simulink model "rst_auto_reg_coupled_tanks_cascade_2018b"  (R2018b)
settings: Solver=FixedStepAuto  StartTime=0.0  StopTime=1000  FixedStep=0.1  RelTol=1e-3
InitFcn:
  | g = 981
  | Km = 3.3
  | Ao1 = 0.17
  | At1 = 15.5528
  | Ao2 = 0.17
  | At2 = 15.5528
  | Ta = 0.1
  | initial_theta = [rand(1,2)]
libraries: dspinverses x4
settings Model: Creator=root  LastModifiedBy=root
settings DataIOCC: SaveFormat=StructureWithTime
settings OptimizationCC: LifeSpan=inf
settings DebuggingCC: LibraryContextMissingDiagnostic=none  SFExecutionAtInitializationDiag=none
settings HardwareCC: ProdBitPerSizeT=32  ProdBitPerPtrDiffT=32  ProdWordSize=32  ProdHWDeviceType=Specified
settings CodeAppCC: StateflowObjectComments=on

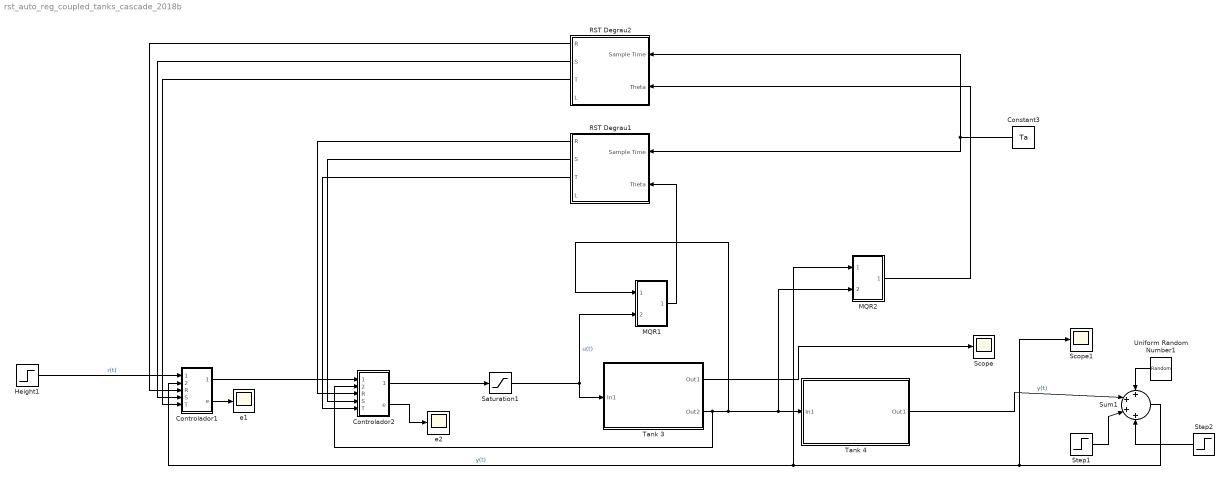
== system rst_auto_reg_coupled_tanks_cascade_2018b ==
  Constant3 : Constant  Value=Ta
  Controlador1 : Subsystem
  Controlador2 : Subsystem
  Height1 : Step  Time=0  After=10  SampleTime=0
  MQR1 : Subsystem
  MQR2 : Subsystem
  RST Degrau1 : Subsystem
  RST Degrau2 : Subsystem
  Saturation1 : Saturate  UpperLimit=12  LowerLimit=-12
  Scope : Scope
  Scope1 : Scope
  Step1 : Step  Time=60  SampleTime=0
  Step2 : Step  Time=61  After=-1  SampleTime=0
  Sum1 : Sum  Inputs=++++
  Tank 3 : Subsystem
  Tank 4 : Subsystem
  Uniform Random Number1 : UniformRandomNumber  Minimum=-0.05  Maximum=0.05  SampleTime=0
  e1 : Scope
  e2 : Scope
  wires:
  Saturation1/1 -> Tank 3/1(In1), MQR1/2("u(t) ")  "u(t)"
  Uniform Random Number1/1 -> Sum1/1
  Step2/1 -> Sum1/4
  Step1/1 -> Sum1/3
  Tank 4/1(Out1) -> Sum1/2  "y(t)"
  Sum1/1 -> Scope1/1, MQR2/1(y(t)), Controlador1/2(y(t))  "y(t)"
  Controlador1/1(u(t)) -> Controlador2/1(r(t))
  Tank 3/2(Out2) -> Controlador2/2(y(t)), MQR1/1(y(t)), MQR2/2("u(t) "), Tank 4/1(In1)
  MQR1/1("Theta(t) ") -> RST Degrau1/2(Theta)
  RST Degrau1/1(R) -> Controlador2/3(R)
  RST Degrau1/2(S) -> Controlador2/4(S)
  RST Degrau1/3(T) -> Controlador2/5(T)
  MQR2/1("Theta(t) ") -> RST Degrau2/2(Theta)
  RST Degrau2/1(R) -> Controlador1/3(R)
  RST Degrau2/2(S) -> Controlador1/4(S)
  RST Degrau2/3(T) -> Controlador1/5(T)
  Height1/1 -> Controlador1/1(r(t))  "r(t)"
  Controlador2/2("e ") -> e2/1
  Controlador2/1(u(t)) -> Saturation1/1
  Controlador1/2("e ") -> e1/1
  Constant3/1 -> RST Degrau1/1(Sample Time), RST Degrau2/1(Sample Time)
  Tank 3/1(Out1) -> Scope/1

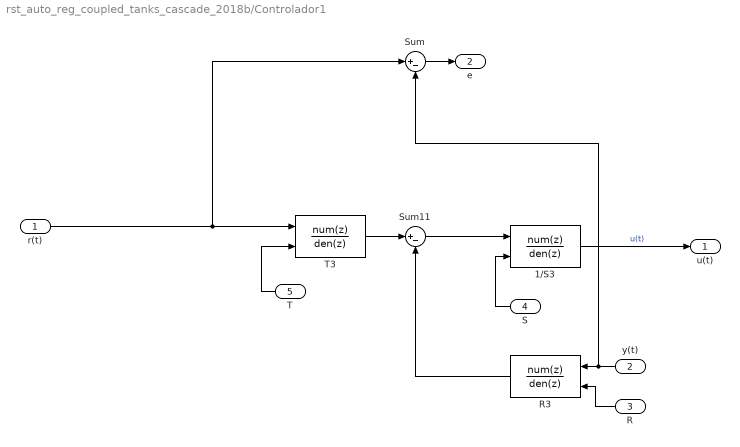
== system rst_auto_reg_coupled_tanks_cascade_2018b/Controlador1 ==
  r(t) : Inport
  y(t) : Inport  Port=2
  R : Inport  Port=3
  S : Inport  Port=4
  T : Inport  Port=5
  1/S3 : DiscreteFilter  Numerator=1  DenominatorSource=Input port  Denominator=1  SampleTime=Ta  a0EqualsOne=on
      settings: InputPortMap=u0,p3
  R3 : DiscreteFilter  NumeratorSource=Input port  Numerator=[-620.2 131.3]  Denominator=1  SampleTime=Ta
      settings: InputPortMap=u0,p1
  Sum : Sum  Inputs=|+-
  Sum11 : Sum  Inputs=|+-
  T3 : DiscreteFilter  NumeratorSource=Input port  Numerator=13.39  Denominator=1  SampleTime=Ta
      settings: InputPortMap=u0,p1
  u(t) : Outport
  "e " : Outport  Port=2
  wires:
  Sum/1 -> "e "/1
  1/S3/1 -> u(t)/1  "u(t)"
  T/1 -> T3/2
  r(t)/1 -> T3/1, Sum/1
  S/1 -> 1/S3/2
  y(t)/1 -> R3/1, Sum/2
  T3/1 -> Sum11/1
  Sum11/1 -> 1/S3/1
  R3/1 -> Sum11/2
  R/1 -> R3/2

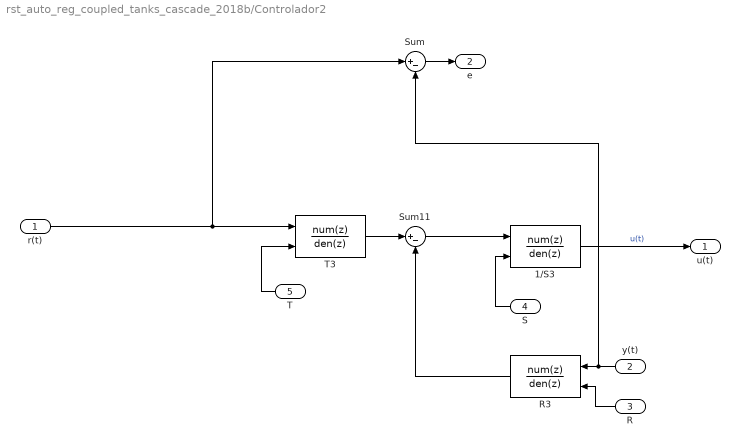
== system rst_auto_reg_coupled_tanks_cascade_2018b/Controlador2 ==
  r(t) : Inport
  y(t) : Inport  Port=2
  R : Inport  Port=3
  S : Inport  Port=4
  T : Inport  Port=5
  1/S3 : DiscreteFilter  Numerator=1  DenominatorSource=Input port  Denominator=1  SampleTime=Ta  a0EqualsOne=on
      settings: InputPortMap=u0,p3
  R3 : DiscreteFilter  NumeratorSource=Input port  Numerator=[-620.2 131.3]  Denominator=1  SampleTime=Ta
      settings: InputPortMap=u0,p1
  Sum : Sum  Inputs=|+-
  Sum11 : Sum  Inputs=|+-
  T3 : DiscreteFilter  NumeratorSource=Input port  Numerator=13.39  Denominator=1  SampleTime=Ta
      settings: InputPortMap=u0,p1
  u(t) : Outport
  "e " : Outport  Port=2
  wires:
  R/1 -> R3/2
  R3/1 -> Sum11/2
  Sum11/1 -> 1/S3/1
  T3/1 -> Sum11/1
  y(t)/1 -> Sum/2, R3/1
  S/1 -> 1/S3/2
  r(t)/1 -> Sum/1, T3/1
  T/1 -> T3/2
  1/S3/1 -> u(t)/1  "u(t)"
  Sum/1 -> "e "/1

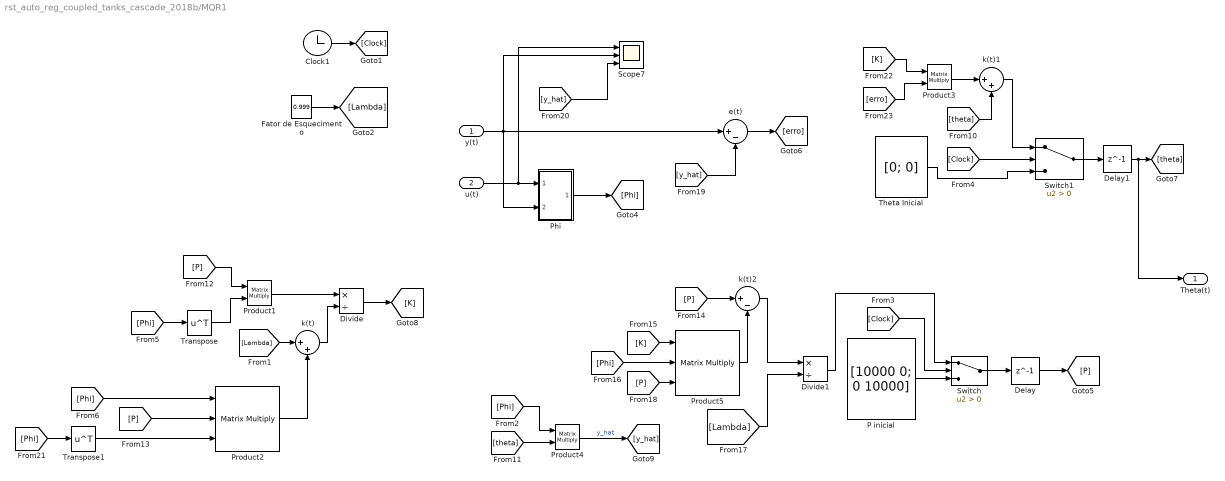
== system rst_auto_reg_coupled_tanks_cascade_2018b/MQR1 ==
  y(t) : Inport
  "u(t) " : Inport  Port=2
  Clock1 : Clock
  Delay : Delay  DelayLength=1  InitialCondition=0
  Delay1 : Delay  DelayLength=1  InitialCondition=0
  Divide : Product  Inputs=*/
  Divide1 : Product  Inputs=*/
  "Fator de Esquecimento " : Constant  Value=0.999
  P inicial : Constant  Value=[10000 0; 0 10000]
  Phi : Subsystem
  Product1 : Product  Multiplication=Matrix(*)
  Product2 : Product  Inputs=3  Multiplication=Matrix(*)
  Product3 : Product  Multiplication=Matrix(*)
  Product4 : Product  Multiplication=Matrix(*)
  Product5 : Product  Inputs=3  Multiplication=Matrix(*)
  Scope7 : Scope  NumInputPorts=3
  Switch : Switch  Criteria=u2 > Threshold
  Switch1 : Switch  Criteria=u2 > Threshold
  "Theta Inicial " : Constant  Value=[0; 0]
  Transpose : Math  Operator=transpose  SaturateOnIntegerOverflow=on
  Transpose1 : Math  Operator=transpose  SaturateOnIntegerOverflow=on
  e(t) : Sum  Inputs=|+-
  k(t) : Sum  Inputs=|++
  k(t)1 : Sum  Inputs=|++
  k(t)2 : Sum  Inputs=|+-
  "Theta(t) " : Outport
  wires:
  Product4/1 -> [y_hat]  "y_hat"
  [Phi] -> Product5/2
  Divide/1 -> [K]
  [Phi] -> Product2/1
  [P] -> Product1/1
  P inicial/1 -> Switch/3
  [K] -> Product5/1
  [y_hat] -> e(t)/2
  [erro] -> Product3/2
  Clock1/1 -> [Clock]
  Transpose/1 -> Product1/2
  [Lambda] -> k(t)/1
  [P] -> Product2/2
  [theta] -> k(t)1/2
  [P] -> k(t)2/1
  [theta] -> Product4/2
  [Clock] -> Switch/2
  [Phi] -> Transpose/1
  Divide1/1 -> Switch/1
  Transpose1/1 -> Product2/3
  "Theta Inicial "/1 -> Switch1/3
  "Fator de Esquecimento "/1 -> [Lambda]
  [P] -> Product5/3
  [Phi] -> Transpose1/1
  Delay/1 -> [P]
  Product3/1 -> k(t)1/1
  e(t)/1 -> [erro]
  Product1/1 -> Divide/1
  [Lambda] -> Divide1/2
  Switch/1 -> Delay/1
  "u(t) "/1 -> Phi/1(u(t)), Scope7/1
  Product5/1 -> k(t)2/2
  Delay1/1 -> [theta], "Theta(t) "/1
  k(t)2/1 -> Divide1/1
  y(t)/1 -> Phi/2(y(t)), Scope7/2, e(t)/1
  [Clock] -> Switch1/2
  Product2/1 -> k(t)/2
  [K] -> Product3/1
  Switch1/1 -> Delay1/1
  [y_hat] -> Scope7/3
  k(t)1/1 -> Switch1/1
  Phi/1(Phi) -> [Phi]
  [Phi] -> Product4/1
  k(t)/1 -> Divide/2

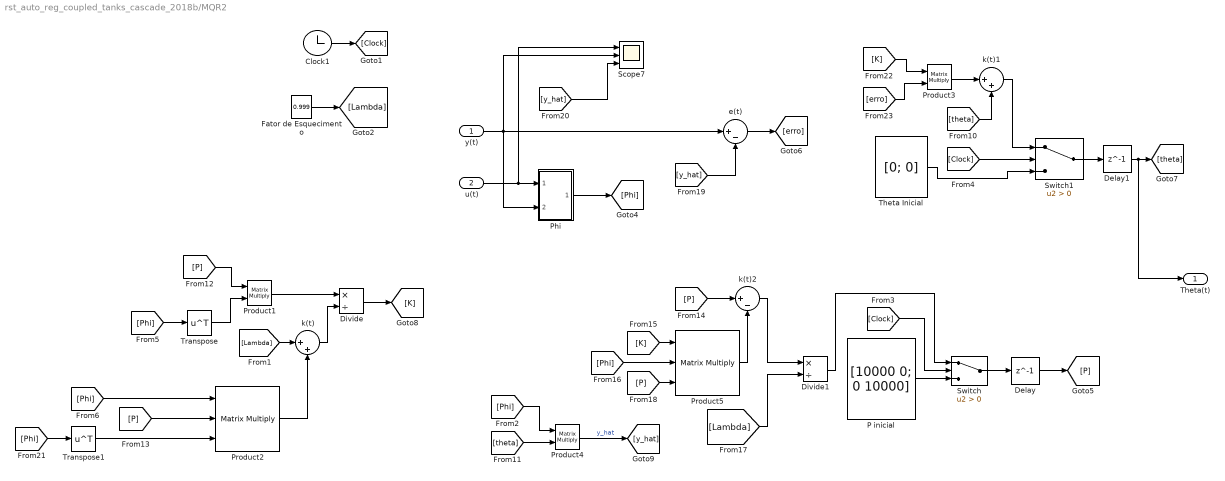
== system rst_auto_reg_coupled_tanks_cascade_2018b/MQR2 ==
  y(t) : Inport
  "u(t) " : Inport  Port=2
  Clock1 : Clock
  Delay : Delay  DelayLength=1  InitialCondition=0
  Delay1 : Delay  DelayLength=1  InitialCondition=0
  Divide : Product  Inputs=*/
  Divide1 : Product  Inputs=*/
  "Fator de Esquecimento " : Constant  Value=0.999
  P inicial : Constant  Value=[10000 0; 0 10000]
  Phi : Subsystem
  Product1 : Product  Multiplication=Matrix(*)
  Product2 : Product  Inputs=3  Multiplication=Matrix(*)
  Product3 : Product  Multiplication=Matrix(*)
  Product4 : Product  Multiplication=Matrix(*)
  Product5 : Product  Inputs=3  Multiplication=Matrix(*)
  Scope7 : Scope  NumInputPorts=3
  Switch : Switch  Criteria=u2 > Threshold
  Switch1 : Switch  Criteria=u2 > Threshold
  "Theta Inicial " : Constant  Value=[0; 0]
  Transpose : Math  Operator=transpose  SaturateOnIntegerOverflow=on
  Transpose1 : Math  Operator=transpose  SaturateOnIntegerOverflow=on
  e(t) : Sum  Inputs=|+-
  k(t) : Sum  Inputs=|++
  k(t)1 : Sum  Inputs=|++
  k(t)2 : Sum  Inputs=|+-
  "Theta(t) " : Outport
  wires:
  k(t)/1 -> Divide/2
  [Phi] -> Product4/1
  Phi/1(Phi) -> [Phi]
  k(t)1/1 -> Switch1/1
  [y_hat] -> Scope7/3
  Switch1/1 -> Delay1/1
  [K] -> Product3/1
  Product2/1 -> k(t)/2
  [Clock] -> Switch1/2
  y(t)/1 -> e(t)/1, Scope7/2, Phi/2(y(t))
  k(t)2/1 -> Divide1/1
  Delay1/1 -> "Theta(t) "/1, [theta]
  Product5/1 -> k(t)2/2
  "u(t) "/1 -> Scope7/1, Phi/1(u(t))
  Switch/1 -> Delay/1
  [Lambda] -> Divide1/2
  Product1/1 -> Divide/1
  e(t)/1 -> [erro]
  Product3/1 -> k(t)1/1
  Delay/1 -> [P]
  [Phi] -> Transpose1/1
  [P] -> Product5/3
  "Fator de Esquecimento "/1 -> [Lambda]
  "Theta Inicial "/1 -> Switch1/3
  Transpose1/1 -> Product2/3
  Divide1/1 -> Switch/1
  [Phi] -> Transpose/1
  [Clock] -> Switch/2
  [theta] -> Product4/2
  [P] -> k(t)2/1
  [theta] -> k(t)1/2
  [P] -> Product2/2
  [Lambda] -> k(t)/1
  Transpose/1 -> Product1/2
  Clock1/1 -> [Clock]
  [erro] -> Product3/2
  [y_hat] -> e(t)/2
  [K] -> Product5/1
  P inicial/1 -> Switch/3
  [P] -> Product1/1
  [Phi] -> Product2/1
  Divide/1 -> [K]
  [Phi] -> Product5/2
  Product4/1 -> [y_hat]  "y_hat"

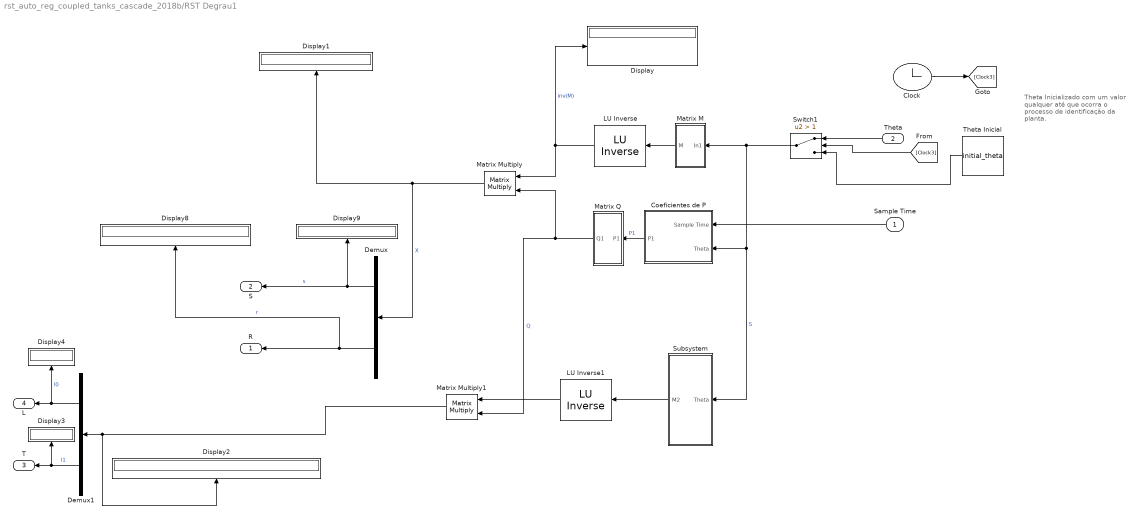
== system rst_auto_reg_coupled_tanks_cascade_2018b/RST Degrau1 ==
  note: Theta Inicializado com um
      | valor qualquer até que ocorra
      |  o processo de identificação
      | da planta.
  Sample Time : Inport
  Theta : Inport  Port=2
  " LU Inverse" : dspinverses/ LU Inverse
      settings: SourceProductName=DSP System Toolbox
  " LU Inverse1" : dspinverses/ LU Inverse
      settings: SourceProductName=DSP System Toolbox
  Clock : Clock
  Coeficientes de P : Subsystem
  Demux : Demux  Outputs=2
  Demux1 : Demux  Outputs=2
  Display{,1..4,8..9} (7 alike) : Display
  Matrix M : Subsystem
  Matrix Multiply : Product  Multiplication=Matrix(*)
  Matrix Multiply1 : Product  Multiplication=Matrix(*)
  Matrix Q : Subsystem
  Subsystem : Subsystem
  Switch1 : Switch  Criteria=u2 > Threshold  Threshold=1
  Theta Inicial : Constant  Value=initial_theta
  R : Outport
  S : Outport  Port=2
  T : Outport  Port=3
  L : Outport  Port=4
  wires:
  Demux/2 -> R/1, Display8/1  "r"
  Demux1/2 -> T/1, Display3/1  "l1"
  Matrix Multiply1/1 -> Demux1/1, Display2/1
  Demux1/1 -> Display4/1, L/1  "l0"
  Subsystem/1(M2) -> " LU Inverse1"/1
  Matrix Q/1(Q1) -> Matrix Multiply/2, Matrix Multiply1/2  "Q"
  " LU Inverse1"/1 -> Matrix Multiply1/1
  Demux/1 -> S/1, Display9/1  "s"
  Matrix M/1(M) -> " LU Inverse"/1
  Theta Inicial/1 -> Switch1/3
  [Clock3] -> Switch1/2
  Theta/1 -> Switch1/1
  Switch1/1 -> Matrix M/1(In1), Subsystem/1(Theta), Coeficientes de P/2(Theta)  "S"
  Clock/1 -> [Clock3]
  Coeficientes de P/1(P1) -> Matrix Q/1(P1)  "P1"
  Sample Time/1 -> Coeficientes de P/1(Sample Time)
  " LU Inverse"/1 -> Display/1, Matrix Multiply/1  "inv(M)"
  Matrix Multiply/1 -> Display1/1, Demux/1  "X"

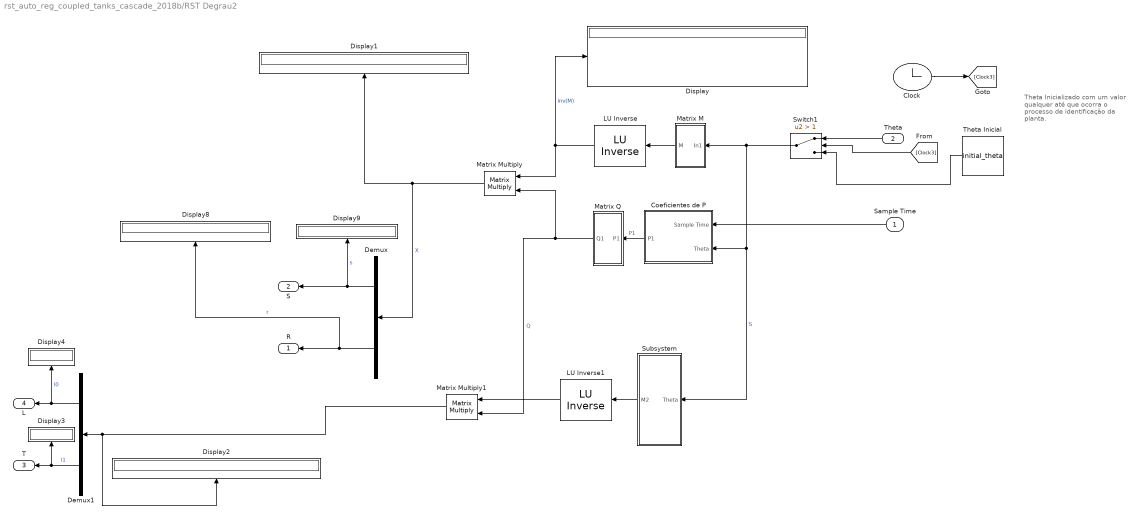
== system rst_auto_reg_coupled_tanks_cascade_2018b/RST Degrau2 ==
  note: Theta Inicializado com um
      | valor qualquer até que ocorra
      |  o processo de identificação
      | da planta.
  Sample Time : Inport
  Theta : Inport  Port=2
  " LU Inverse" : dspinverses/ LU Inverse
      settings: SourceProductName=DSP System Toolbox
  " LU Inverse1" : dspinverses/ LU Inverse
      settings: SourceProductName=DSP System Toolbox
  Clock : Clock
  Coeficientes de P : Subsystem
  Demux : Demux  Outputs=2
  Demux1 : Demux  Outputs=2
  Display{,1..4,8..9} (7 alike) : Display
  Matrix M : Subsystem
  Matrix Multiply : Product  Multiplication=Matrix(*)
  Matrix Multiply1 : Product  Multiplication=Matrix(*)
  Matrix Q : Subsystem
  Subsystem : Subsystem
  Switch1 : Switch  Criteria=u2 > Threshold  Threshold=1
  Theta Inicial : Constant  Value=initial_theta
  R : Outport
  S : Outport  Port=2
  T : Outport  Port=3
  L : Outport  Port=4
  wires:
  Matrix Multiply/1 -> Demux/1, Display1/1  "X"
  " LU Inverse"/1 -> Matrix Multiply/1, Display/1  "inv(M)"
  Sample Time/1 -> Coeficientes de P/1(Sample Time)
  Coeficientes de P/1(P1) -> Matrix Q/1(P1)  "P1"
  Clock/1 -> [Clock3]
  Switch1/1 -> Subsystem/1(Theta), Coeficientes de P/2(Theta), Matrix M/1(In1)  "S"
  Theta/1 -> Switch1/1
  [Clock3] -> Switch1/2
  Theta Inicial/1 -> Switch1/3
  Matrix M/1(M) -> " LU Inverse"/1
  Demux/1 -> S/1, Display9/1  "s"
  " LU Inverse1"/1 -> Matrix Multiply1/1
  Matrix Q/1(Q1) -> Matrix Multiply1/2, Matrix Multiply/2  "Q"
  Subsystem/1(M2) -> " LU Inverse1"/1
  Demux1/1 -> L/1, Display4/1  "l0"
  Matrix Multiply1/1 -> Display2/1, Demux1/1
  Demux1/2 -> Display3/1, T/1  "l1"
  Demux/2 -> R/1, Display8/1  "r"

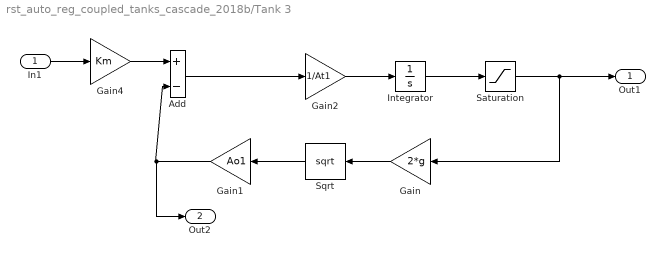
== system rst_auto_reg_coupled_tanks_cascade_2018b/Tank 3 ==
  In1 : Inport
  Add : Sum  Inputs=+-
  Gain : Gain  Gain=2*g
  Gain1 : Gain  Gain=Ao1
  Gain2 : Gain  Gain=1/At1
  Gain4 : Gain  Gain=Km
  Integrator : Integrator
  Saturation : Saturate  UpperLimit=30  LowerLimit=0
  Sqrt : Sqrt  SaturateOnIntegerOverflow=on
  Out1 : Outport
  Out2 : Outport  Port=2
  wires:
  Gain4/1 -> Add/1
  Add/1 -> Gain2/1
  Saturation/1 -> Gain/1, Out1/1
  Integrator/1 -> Saturation/1
  Sqrt/1 -> Gain1/1
  In1/1 -> Gain4/1
  Gain/1 -> Sqrt/1
  Gain1/1 -> Add/2, Out2/1
  Gain2/1 -> Integrator/1

== system rst_auto_reg_coupled_tanks_cascade_2018b/Tank 4 ==
  In1 : Inport
  Add1 : Sum  Inputs=+-
  Gain4 : Gain  Gain=2*g
  Gain5 : Gain  Gain=Ao2
  Gain6 : Gain  Gain=1/At2
  Integrator1 : Integrator
  Saturation : Saturate  UpperLimit=30  LowerLimit=0
  Sqrt1 : Sqrt  SaturateOnIntegerOverflow=on
  Out1 : Outport
  wires:
  Saturation/1 -> Gain4/1, Out1/1
  Gain5/1 -> Add1/2
  Integrator1/1 -> Saturation/1
  Gain4/1 -> Sqrt1/1
  Sqrt1/1 -> Gain5/1
  In1/1 -> Add1/1
  Gain6/1 -> Integrator1/1
  Add1/1 -> Gain6/1

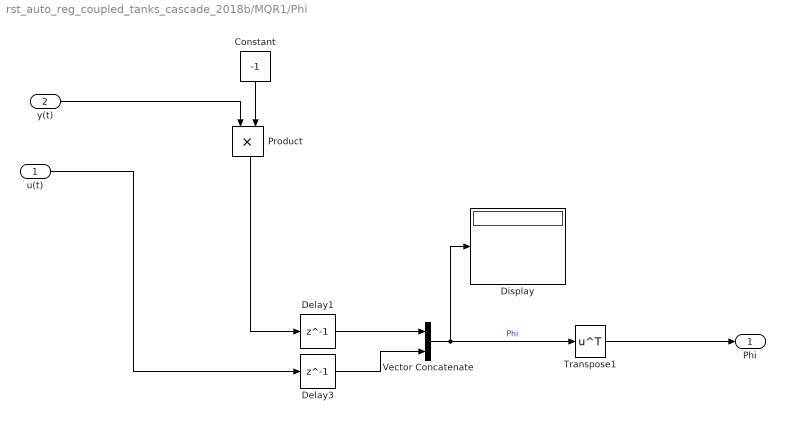
== system rst_auto_reg_coupled_tanks_cascade_2018b/MQR1/Phi ==
  u(t) : Inport
  y(t) : Inport  Port=2
  Constant : Constant  Value=-1
  Delay1 : Delay  DelayLength=1
  Delay3 : Delay  DelayLength=1
  Display : Display
  Product : Product
  Transpose1 : Math  Operator=transpose  SaturateOnIntegerOverflow=on
  Vector Concatenate : Concatenate
  Phi : Outport
  wires:
  Constant/1 -> Product/2
  Transpose1/1 -> Phi/1
  Delay1/1 -> Vector Concatenate/1
  Delay3/1 -> Vector Concatenate/2
  y(t)/1 -> Product/1
  Product/1 -> Delay1/1
  Vector Concatenate/1 -> Display/1, Transpose1/1  "Phi"
  u(t)/1 -> Delay3/1

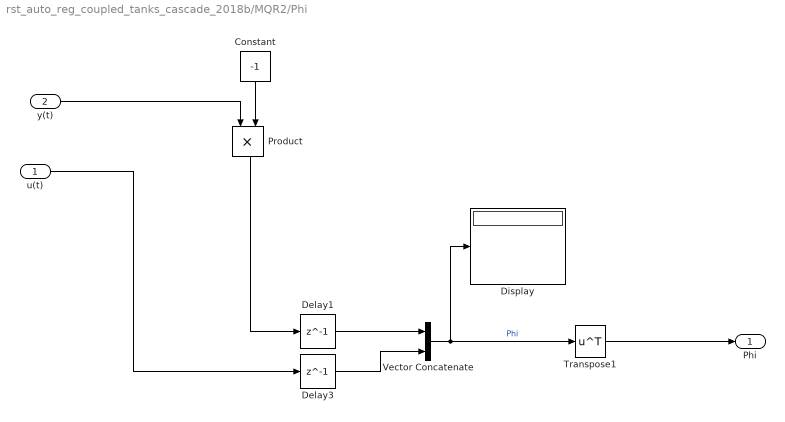
== system rst_auto_reg_coupled_tanks_cascade_2018b/MQR2/Phi ==
  u(t) : Inport
  y(t) : Inport  Port=2
  Constant : Constant  Value=-1
  Delay1 : Delay  DelayLength=1
  Delay3 : Delay  DelayLength=1
  Display : Display
  Product : Product
  Transpose1 : Math  Operator=transpose  SaturateOnIntegerOverflow=on
  Vector Concatenate : Concatenate
  Phi : Outport
  wires:
  u(t)/1 -> Delay3/1
  Vector Concatenate/1 -> Transpose1/1, Display/1  "Phi"
  Product/1 -> Delay1/1
  y(t)/1 -> Product/1
  Delay3/1 -> Vector Concatenate/2
  Delay1/1 -> Vector Concatenate/1
  Transpose1/1 -> Phi/1
  Constant/1 -> Product/2

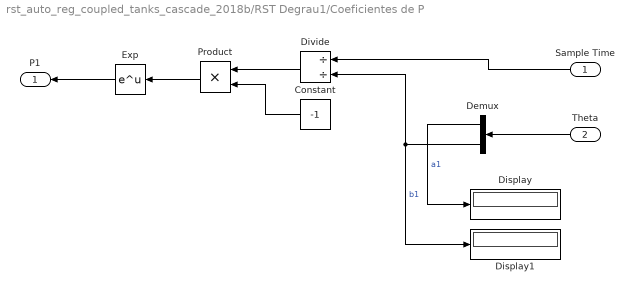
== system rst_auto_reg_coupled_tanks_cascade_2018b/RST Degrau1/Coeficientes de P ==
  Sample Time : Inport
  Theta : Inport  Port=2
  Constant : Constant  Value=-1
  Demux : Demux  Outputs=2
  Display : Display
  Display1 : Display
  Divide : Product  Inputs=//
  Exp : Math  SaturateOnIntegerOverflow=on
  Product : Product
  P1 : Outport
  wires:
  Exp/1 -> P1/1
  Product/1 -> Exp/1
  Constant/1 -> Product/2
  Divide/1 -> Product/1
  Sample Time/1 -> Divide/1
  Demux/2 -> Display1/1, Divide/2  "b1"
  Demux/1 -> Display/1  "a1"
  Theta/1 -> Demux/1

== system rst_auto_reg_coupled_tanks_cascade_2018b/RST Degrau1/Matrix M ==
  In1 : Inport
  " 1" : Constant  Value=0
  2 : Constant
  Demux : Demux  Outputs=2
  Display1 : Display
  Matrix Concatenate12 : Concatenate  Mode=Multidimensional array
  Matrix Concatenate6 : Concatenate  Mode=Multidimensional array  ConcatenateDimension=2
  Matrix Concatenate9 : Concatenate  Mode=Multidimensional array  ConcatenateDimension=2
  M : Outport
  wires:
  Demux/2 -> Matrix Concatenate9/2  "b1"
  Demux/1 -> Matrix Concatenate9/1  "a1"
  Matrix Concatenate12/1 -> Display1/1, M/1
  Matrix Concatenate9/1 -> Matrix Concatenate12/2
  Matrix Concatenate6/1 -> Matrix Concatenate12/1
  " 1"/1 -> Matrix Concatenate6/2
  2/1 -> Matrix Concatenate6/1  "1"
  In1/1 -> Demux/1

== system rst_auto_reg_coupled_tanks_cascade_2018b/RST Degrau1/Matrix Q ==
  P1 : Inport
  Constant : Constant
  Display1 : Display
  Matrix Concatenate1 : Concatenate  Mode=Multidimensional array
  Q1 : Outport
  wires:
  Constant/1 -> Matrix Concatenate1/1
  P1/1 -> Matrix Concatenate1/2
  Matrix Concatenate1/1 -> Display1/1, Q1/1

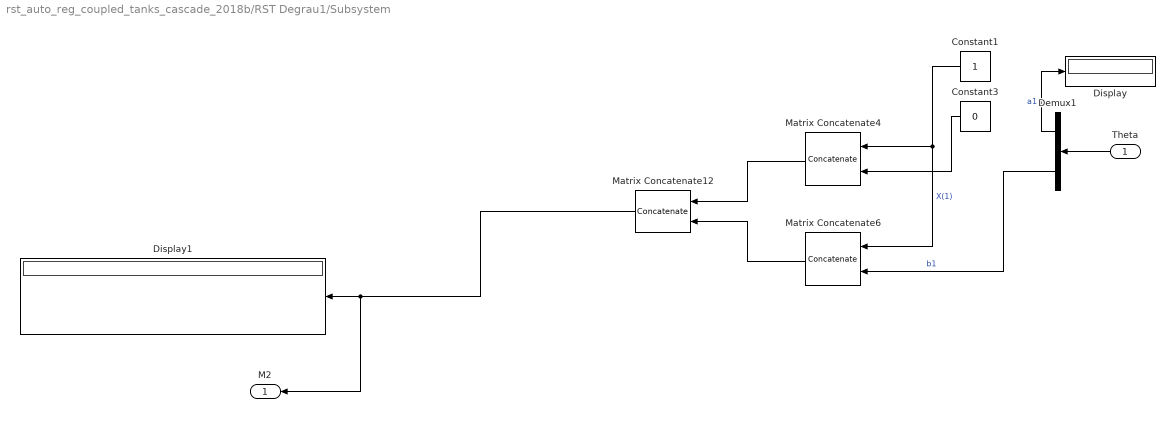
== system rst_auto_reg_coupled_tanks_cascade_2018b/RST Degrau1/Subsystem ==
  Theta : Inport
  Constant1 : Constant
  Constant3 : Constant  Value=0
  Demux1 : Demux  Outputs=2
  Display : Display
  Display1 : Display
  Matrix Concatenate12 : Concatenate  Mode=Multidimensional array
  Matrix Concatenate4 : Concatenate  Mode=Multidimensional array  ConcatenateDimension=2
  Matrix Concatenate6 : Concatenate  Mode=Multidimensional array  ConcatenateDimension=2
  M2 : Outport
  wires:
  Demux1/1 -> Display/1  "a1"
  Demux1/2 -> Matrix Concatenate6/2  "b1"
  Matrix Concatenate4/1 -> Matrix Concatenate12/1
  Constant3/1 -> Matrix Concatenate4/2
  Constant1/1 -> Matrix Concatenate4/1, Matrix Concatenate6/1  "X(1)"
  Theta/1 -> Demux1/1
  Matrix Concatenate6/1 -> Matrix Concatenate12/2
  Matrix Concatenate12/1 -> M2/1, Display1/1

== system rst_auto_reg_coupled_tanks_cascade_2018b/RST Degrau2/Coeficientes de P ==
  Sample Time : Inport
  Theta : Inport  Port=2
  Constant : Constant  Value=-1
  Demux : Demux  Outputs=2
  Display : Display
  Display1 : Display
  Divide : Product  Inputs=//
  Exp : Math  SaturateOnIntegerOverflow=on
  Product : Product
  P1 : Outport
  wires:
  Theta/1 -> Demux/1
  Demux/1 -> Display/1  "a1"
  Demux/2 -> Divide/2, Display1/1  "b1"
  Sample Time/1 -> Divide/1
  Divide/1 -> Product/1
  Constant/1 -> Product/2
  Product/1 -> Exp/1
  Exp/1 -> P1/1

== system rst_auto_reg_coupled_tanks_cascade_2018b/RST Degrau2/Matrix M ==
  In1 : Inport
  " 1" : Constant  Value=0
  2 : Constant
  Demux : Demux  Outputs=2
  Display1 : Display
  Matrix Concatenate12 : Concatenate  Mode=Multidimensional array
  Matrix Concatenate6 : Concatenate  Mode=Multidimensional array  ConcatenateDimension=2
  Matrix Concatenate9 : Concatenate  Mode=Multidimensional array  ConcatenateDimension=2
  M : Outport
  wires:
  In1/1 -> Demux/1
  2/1 -> Matrix Concatenate6/1  "1"
  " 1"/1 -> Matrix Concatenate6/2
  Matrix Concatenate6/1 -> Matrix Concatenate12/1
  Matrix Concatenate9/1 -> Matrix Concatenate12/2
  Matrix Concatenate12/1 -> M/1, Display1/1
  Demux/1 -> Matrix Concatenate9/1  "a1"
  Demux/2 -> Matrix Concatenate9/2  "b1"

== system rst_auto_reg_coupled_tanks_cascade_2018b/RST Degrau2/Matrix Q ==
  P1 : Inport
  Constant : Constant
  Display1 : Display
  Matrix Concatenate1 : Concatenate  Mode=Multidimensional array
  Q1 : Outport
  wires:
  Matrix Concatenate1/1 -> Q1/1, Display1/1
  P1/1 -> Matrix Concatenate1/2
  Constant/1 -> Matrix Concatenate1/1

== system rst_auto_reg_coupled_tanks_cascade_2018b/RST Degrau2/Subsystem ==
  Theta : Inport
  Constant1 : Constant
  Constant3 : Constant  Value=0
  Demux1 : Demux  Outputs=2
  Display : Display
  Display1 : Display
  Matrix Concatenate12 : Concatenate  Mode=Multidimensional array
  Matrix Concatenate4 : Concatenate  Mode=Multidimensional array  ConcatenateDimension=2
  Matrix Concatenate6 : Concatenate  Mode=Multidimensional array  ConcatenateDimension=2
  M2 : Outport
  wires:
  Matrix Concatenate6/1 -> Matrix Concatenate12/2
  Theta/1 -> Demux1/1
  Constant1/1 -> Matrix Concatenate6/1, Matrix Concatenate4/1  "X(1)"
  Constant3/1 -> Matrix Concatenate4/2
  Matrix Concatenate4/1 -> Matrix Concatenate12/1
  Demux1/2 -> Matrix Concatenate6/2  "b1"
  Demux1/1 -> Display/1  "a1"
  Matrix Concatenate12/1 -> Display1/1, M2/1
